simulink model "on_of"  (R2019a)
settings: Solver=VariableStepAuto  StartTime=0.0  StopTime=1500  RelTol=1e-3
settings Model: Creator=josefernandorosaribeiro  LastModifiedBy=josefernandorosaribeiro

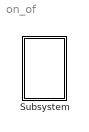
== system on_of ==
  Subsystem : Subsystem

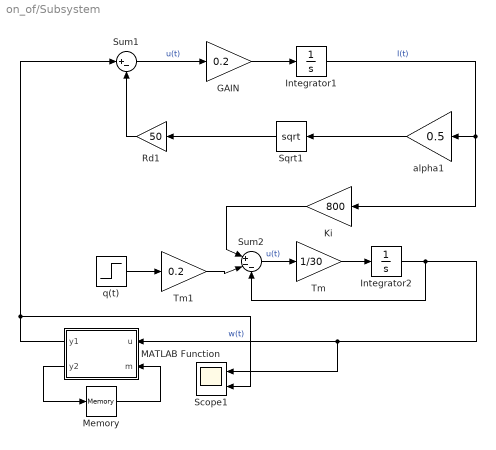
== system on_of/Subsystem ==
  GAIN : Gain  Gain=0.2
  Integrator1 : Integrator  InitialCondition=0.0072
  Integrator2 : Integrator  InitialCondition=15
  Ki : Gain  Gain=800
  MATLAB Function : MATLAB Function  TreatAsAtomicUnit=on
  Memory : Memory  InitialCondition=1
  Rd1 : Gain  Gain=50
  Scope1 : Scope  NumInputPorts=2
  Sqrt1 : Sqrt  SaturateOnIntegerOverflow=on
  Sum1 : Sum  Inputs=|+-
  Sum2 : Sum  Inputs=|+--
  Tm : Gain  Gain=1/30
  Tm1 : Gain  Gain=0.2
  alpha1 : Gain  Gain=0.5
  q(t) : Step  Before=1  SampleTime=0
  wires:
  Tm1/1 -> Sum2/2
  q(t)/1 -> Tm1/1
  Sqrt1/1 -> Rd1/1
  Sum2/1 -> Tm/1  "u(t)"
  GAIN/1 -> Integrator1/1
  Ki/1 -> Sum2/1
  Tm/1 -> Integrator2/1
  Integrator2/1 -> Sum2/3, MATLAB Function/1(u), Scope1/1  "w(t)"
  Rd1/1 -> Sum1/2
  alpha1/1 -> Sqrt1/1
  MATLAB Function/1(y1) -> Sum1/1, Scope1/2
  Integrator1/1 -> Ki/1, alpha1/1  "I(t)"
  Sum1/1 -> GAIN/1  "u(t)"
  MATLAB Function/2(y2) -> Memory/1
  Memory/1 -> MATLAB Function/2(m)

== matlab function on_of/Subsystem/MATLAB Function ==
  data: u input; y1 output; y2 output; m input
function [y1, y2]= fcn(u, m)

lower_bound = 5;
upper_bound = 15;
active = m;
if active
    y1 = 5;
else
    y1 = 1;
end

if u>=upper_bound
    active = 0;
elseif u<=lower_bound
    active = 1;
end
y2 = active;
